simulink model "ex"  (R2014a)
settings: Solver=ode45  StartTime=0.0  StopTime=20.0  RelTol=1e-3
settings Model: Creator=root  LastModifiedBy=root

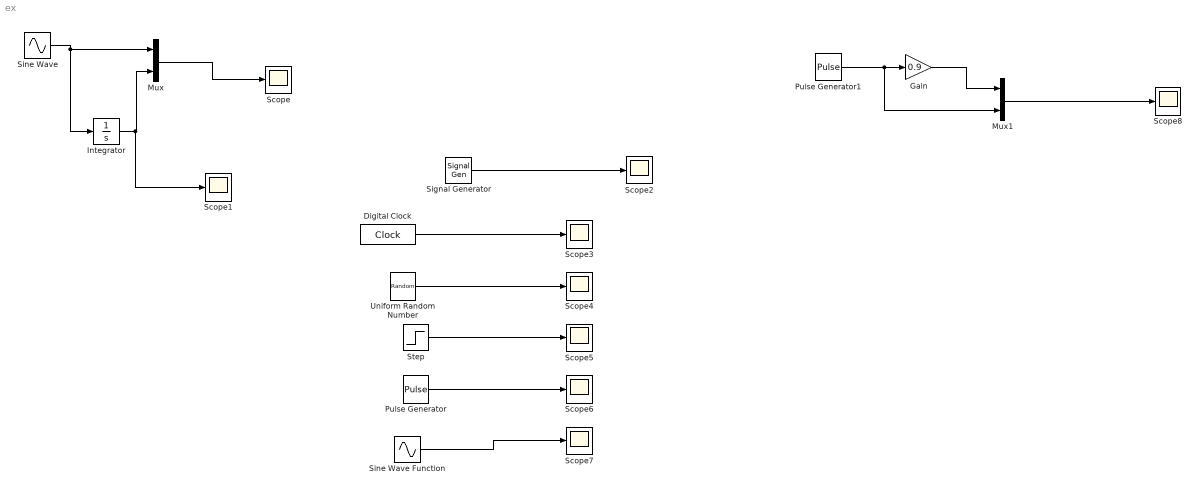
== system ex ==
  Digital Clock : DigitalClock
  Gain : Gain  Gain=0.9
  Integrator : Integrator
  Mux : Mux  Inputs=2
  Mux1 : Mux  Inputs=2
  Pulse Generator : DiscretePulseGenerator  PulseType=Time based  Period=10  PulseWidth=5
  Pulse Generator1 : DiscretePulseGenerator  PulseType=Time based  Amplitude=0.7  Period=1  PulseWidth=50
  Scope{,1..8} (9 alike) : Scope
      Scope2 settings: SaveName=ScopeData2
      Scope3 settings: SaveName=ScopeData3
      Scope4 settings: SaveName=ScopeData4
      Scope5 settings: SaveName=ScopeData5
      Scope6 settings: SaveName=ScopeData6
      Scope7 settings: SaveName=ScopeData7
      Scope8 settings: SaveName=ScopeData8
  Signal Generator : SignalGenerator  WaveForm=random  Units=rad/sec
  Sine Wave : Sin  Phase=45  SampleTime=0
  Sine Wave Function : Sin  TimeSource=Use external signal  SampleTime=0
  Step : Step  SampleTime=0
  Uniform Random Number : UniformRandomNumber  Minimum=-2  SampleTime=0.3
  wires:
  Sine Wave/1 -> Mux/1, Integrator/1
  Integrator/1 -> Scope1/1, Mux/2
  Mux/1 -> Scope/1
  Signal Generator/1 -> Scope2/1
  Digital Clock/1 -> Scope3/1
  Uniform Random Number/1 -> Scope4/1
  Step/1 -> Scope5/1
  Pulse Generator/1 -> Scope6/1
  Sine Wave Function/1 -> Scope7/1
  Gain/1 -> Mux1/1
  Pulse Generator1/1 -> Mux1/2, Gain/1
  Mux1/1 -> Scope8/1
